simulink model "Damn"  (R2022b)
settings: Solver=VariableStepAuto  StartTime=0.0  StopTime=10.0  RelTol=1e-3
values from neighbouring files (symbols this model uses):
  A = [0 1; -3 -5]    [Session.m]    (also in Session_1.m = [0 1 0;0 0 1;-1 -5 -6])
  B = [0 1]'    [Session.m]    (also in Session_1.m = [0 0 1]')
  C = [1 0]    [Session.m]    (also in Session_1.m)
  D = [0]    [Session.m]    (also in Session_1.m)
  K = [180.11, 11]    [Session.m]    (also in Session_1.m = place(A, B, J))
settings Model: Creator=adlercohen  LastModifiedBy=adlercohen

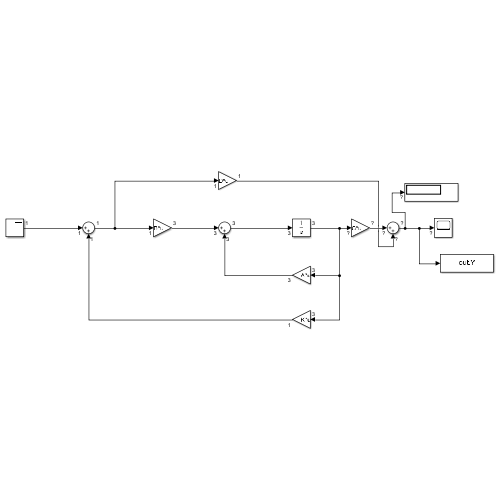
[thumbnail: Simulink's stored preview of the top-level diagram]
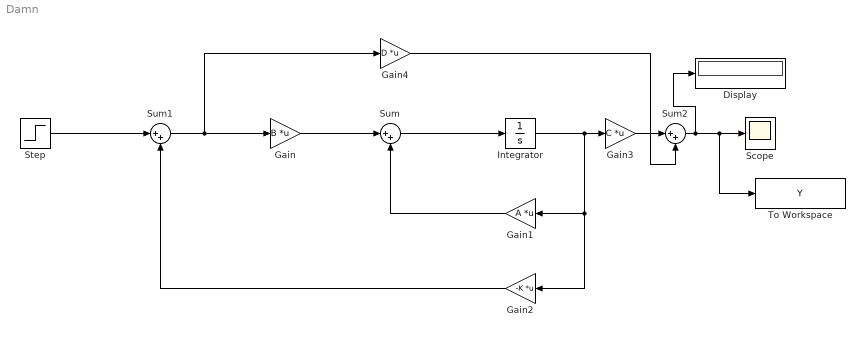
== system Damn ==
  Display : Display
  Gain : Gain  Gain=B  Multiplication=Matrix(K*u)
  Gain1 : Gain  Gain=A  Multiplication=Matrix(K*u)
  Gain2 : Gain  Gain=-K  Multiplication=Matrix(K*u)
  Gain3 : Gain  Gain=C  Multiplication=Matrix(K*u)
  Gain4 : Gain  Gain=D  Multiplication=Matrix(K*u)
  Integrator : Integrator
  Scope : Scope
  Step : Step  Time=0  SampleTime=0
  Sum : Sum  Inputs=|++
  Sum1 : Sum  Inputs=|++
  Sum2 : Sum  Inputs=|++
  To Workspace : ToWorkspace  VariableName=Y  SampleTime=-1
  wires:
  Gain4/1 -> Sum2/2
  Sum2/1 -> Display/1, To Workspace/1, Scope/1
  Step/1 -> Sum1/1
  Gain3/1 -> Sum2/1
  Gain1/1 -> Sum/2
  Integrator/1 -> Gain2/1, Gain1/1, Gain3/1
  Gain/1 -> Sum/1
  Gain2/1 -> Sum1/2
  Sum1/1 -> Gain4/1, Gain/1
  Sum/1 -> Integrator/1
